simulink model "ASK"  (R2021b)
settings: Solver=VariableStepAuto  StartTime=0.0  StopTime=30  RelTol=1e-3
libraries: commrandsrc3 x1
settings Model: Creator=zhang  LastModifiedBy=zhang
settings SolverCC: AlgebraicLoopSolver=TrustRegion
settings DebuggingCC: SFMachineParentedDataDiag=warning

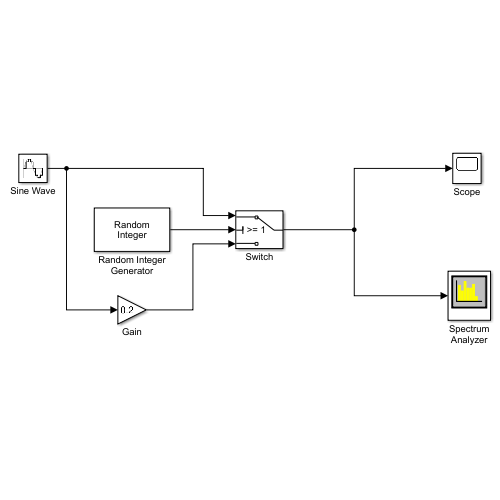
[thumbnail: Simulink's stored preview of the top-level diagram]
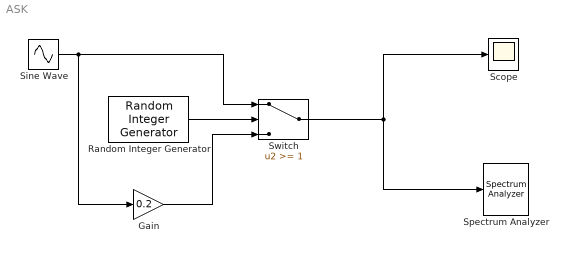
== system ASK ==
  Gain : Gain  Gain=0.2
  Random Integer Generator : commrandsrc3/Random Integer Generator  SetSize=2  SeedSource=Auto  Seed=0  SampleTime=1  SamplesPerFrame=1  OutputDataType=single  SimulateUsing=Code generation
  Scope : Scope
  Sine Wave : Sin  Frequency=2*pi*10  SampleTime=1/100
  Spectrum Analyzer : SpectrumAnalyzer
  Switch : Switch  Threshold=1
  wires:
  Random Integer Generator/1 -> Switch/2
  Switch/1 -> Scope/1, Spectrum Analyzer/1
  Sine Wave/1 -> Gain/1, Switch/1
  Gain/1 -> Switch/3
